simulink model "Controlador_de_corriente_v5"  (R2014b)
settings: Solver=VariableStepAuto  StartTime=0.0  StopTime=50e-3  RelTol=1e-3
settings Model: Creator=juanm  LastModifiedBy=Javi
settings DataIOCC: LimitDataPoints=off  SaveFormat=Dataset
settings OptimizationCC: UseDivisionForNetSlopeComputation=off  LifeSpan=auto  SimCompilerOptimization=off
settings DebuggingCC: SolverPrmCheckMsg=none  FcnCallInpInsideContextMsg=error  FrameProcessingCompatibilityMsg=error  SFUnexpectedBacktrackingDiag=error  SFNoUnconditionalDefaultTransitionDiag=error
settings HardwareCC: ProdBitPerPointer=64  ProdLargestAtomicFloat=Float  ProdIntDivRoundTo=Zero  ProdEndianess=LittleEndian  ProdWordSize=64  ProdHWDeviceType=Intel->x86-64 (Windows64)
settings ModelReferenceCC: PropagateSignalLabelsOutOfModel=on
settings RTWCC: RTWCompilerOptimization=off
settings GRTTargetCC: TargetLangStandard=C99 (ISO)  GeneratePreprocessorConditionals=Use local settings
settings ConfigurationSet: Description=Simscape Multibody

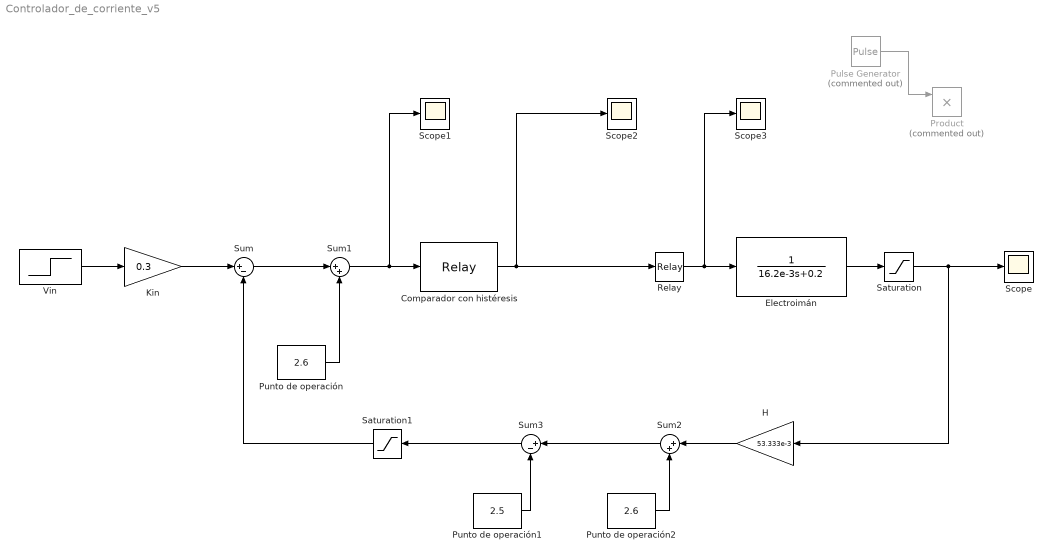
== system Controlador_de_corriente_v5 ==
  Comparador con histéresis : Relay  OnSwitchValue=2.5125  OffSwitchValue=2.4875  OnOutputValue=5
  Electroimán : TransferFcn  Denominator=[16.2e-3 0.2]
  H : Gain  Gain=53.333e-3
  Kin : Gain  Gain=0.3
  Product : Product  Commented=on
  Pulse Generator : DiscretePulseGenerator  Commented=on  PulseType=Time based  Period=40e-6  PulseWidth=10
  Punto de operación : Constant  Value=2.6
  Punto de operación1 : Constant  Value=2.5
  Punto de operación2 : Constant  Value=2.6
  Relay : Relay  OnSwitchValue=3  OffSwitchValue=2  OnOutputValue=24  OffOutputValue=-24
  Saturation : Saturate  UpperLimit=40  LowerLimit=-40
  Saturation1 : Saturate  UpperLimit=5  LowerLimit=0
  Scope{,1..3} (4 alike) : Scope
      Scope settings: TimeRange=0.003567149833283473  YMin=-0.2  YMax=0.4000000000000001
      Scope1 settings: YMin=2.725  YMax=3.475
      Scope2 settings: TimeRange=0.002665873959571937  YMin=-30  YMax=30  SaveName=ScopeData2
      Scope3 settings: YMin=-30.00000  YMax=30.00000  SaveName=ScopeData3
  Sum : Sum  Inputs=|+-
  Sum1 : Sum  Inputs=|++
  Sum2 : Sum  Inputs=|++
  Sum3 : Sum  Inputs=|+-
  Vin : Step  Time=1e-6  SampleTime=0
  wires:
  Comparador con histéresis/1 -> Relay/1, Scope2/1
  Kin/1 -> Sum/1
  Electroimán/1 -> Saturation/1
  Saturation/1 -> H/1, Scope/1
  Pulse Generator/1 -> Product/1
  Relay/1 -> Scope3/1, Electroimán/1
  Sum/1 -> Sum1/1
  Sum1/1 -> Scope1/1, Comparador con histéresis/1
  Punto de operación/1 -> Sum1/2
  H/1 -> Sum2/1
  Sum2/1 -> Sum3/1
  Punto de operación2/1 -> Sum2/2
  Punto de operación1/1 -> Sum3/2
  Sum3/1 -> Saturation1/1
  Saturation1/1 -> Sum/2
  Vin/1 -> Kin/1
